simulink model "LR90x2D101"  (R2024a)
settings: Solver=VariableStepAuto  StartTime=0.0  StopTime=10.0  RelTol=1e-3
PreLoadFcn:
  | boiler_simulink=readfis('C:\Users\nagal\OneDrive\Рабочий стол\Boiler.fis');
libraries: fuzblock x1
settings Model: Creator=Jakepps  LastModifiedBy=kiril
settings SolverCC: AlgebraicLoopSolver=TrustRegion
settings DataIOCC: LimitDataPoints=on  SaveOutput=off  SaveTime=off
settings OptimizationCC: BlockReduction=off  BooleanDataType=off  LifeSpan=inf
settings DebuggingCC: SaveWithParameterizedLinksMsg=none  UnderspecifiedInitializationDetection=Classic  MergeDetectMultiDrivingBlocksExec=none  SignalResolutionControl=TryResolveAllWithWarning  UnconnectedInputMsg=warning  UnconnectedOutputMsg=warning  UnconnectedLineMsg=warning  AllowSymbolicDim=off  SFUnexpectedBacktrackingDiag=warning  SFNoUnconditionalDefaultTransitionDiag=warning  SFExecutionAtInitializationDiag=none  ArithmeticOperatorsInVariantConditions=warning
settings HardwareCC: TargetUnknown=on
settings ModelReferenceCC: EnableRefExpFcnMdlSchedulingChecks=on
settings SFSimCC: SimUseLocalCustomCode=off  CustomCodeUndefinedFunction=UseInterfaceOnly
settings RTWCC: RTWUseLocalCustomCode=off  GPUComputeCapability=3.5
settings CodeAppCC: StateflowObjectComments=on
settings GRTTargetCC: TargetLangStandard=C89/C90 (ANSI)

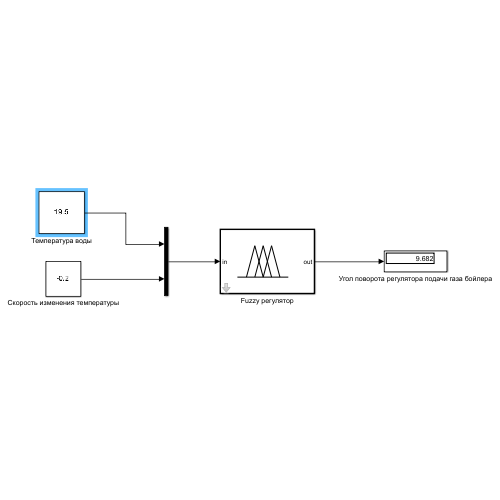
[thumbnail: Simulink's stored preview of the top-level diagram]
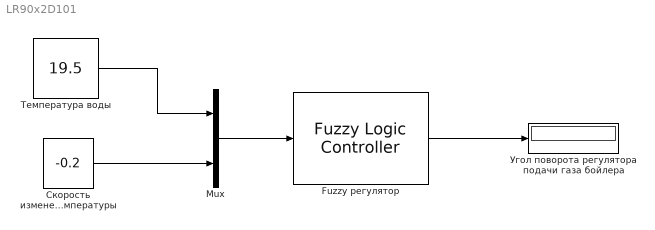
== system LR90x2D101 ==
  Fuzzy регулятор : fuzblock/Fuzzy Logic  Controller  FIS='C:\Users\kiril\OneDrive\Рабочий стол\нейронки\fuzzyMat\lab9-10\Boiler.fis'  OutputSampleNumber=101  DataType=double  FuzzifiedInputs=off  RuleFiringStrengths=off  RuleOutputs=off  AggregatedOutputs=off  SimulateUsing=Interpreted execution  OutOfRangeInputValueMessage=warning  NoRuleFiredMessage=warning  EmptyOutputFuzzySetMessage=warning
  Mux : Mux  Inputs=2
  Скорость изменения температуры : Constant  Value=-0.2
  Температура воды : Constant  Value=19.5
  Угол поворота регулятора подачи газа бойлера : Display
  wires:
  Скорость изменения температуры/1 -> Mux/2
  Mux/1 -> Fuzzy регулятор/1
  Fuzzy регулятор/1 -> Угол поворота регулятора подачи газа бойлера/1
  Температура воды/1 -> Mux/1
